simulink model "lab-6-simulink"  (R2018a)
settings: Solver=ode23t  StartTime=0.0  StopTime=10.0  RelTol=1e-3
values from neighbouring files (symbols this model uses):
  Kd = 0    [lab-6-q1.m]    (also in lab-6-q2.m; lab-6-q3.m = 10)
  Ki = 0    [lab-6-q1.m]    (also in lab-6-q2.m = 15; lab-6-q3.m = 5)
  Kp = 40    [lab-6-q1.m]    (also in lab-6-q2.m = 5; lab-6-q3.m = 5)
libraries: simulink x1
settings Model: Creator=katherto  LastModifiedBy=katherto

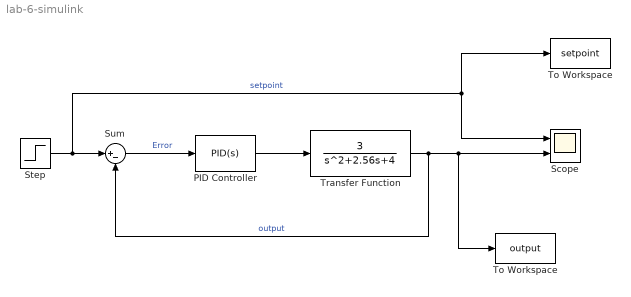
== system lab-6-simulink ==
  "PID Controller  " : simulink/Continuous/PID Controller  Controller=PID  TimeDomain=Continuous-time  SampleTime=-1  IntegratorMethod=Forward Euler  FilterMethod=Forward Euler  Form=Parallel  UseFilter=on  ControllerParametersSource=internal  P=Kp  I=Ki  D=Kd  N=100  InitialConditionSource=internal  InitialConditionForIntegrator=0  InitialConditionForFilter=0  ExternalReset=none  LimitOutput=off  UpperSaturationLimit=inf  LowerSaturationLimit=-inf  LinearizeAsGain=on  AntiWindupMode=none  Kb=1  TrackingMode=off  Kt=1  PParamMin=[]  PParamMax=[]  IParamMin=[]  IParamMax=[]  DParamMin=[]  DParamMax=[]  NParamMin=[]  NParamMax=[]  KbParamMin=[]  KbParamMax=[]  KtParamMin=[]  KtParamMax=[]  POutMin=[]  POutMax=[]  IOutMin=[]  IOutMax=[]  DOutMin=[]  DOutMax=[]  NOutMin=[]  NOutMax=[]  KbOutMin=[]  KbOutMax=[]  KtOutMin=[]  KtOutMax=[]  IntegratorOutMin=[]  IntegratorOutMax=[]  FilterOutMin=[]  FilterOutMax=[]  SumOutMin=[]  SumOutMax=[]  SumI1OutMin=[]  SumI1OutMax=[]  SumI2OutMin=[]  SumI2OutMax=[]  SumI3OutMin=[]  SumI3OutMax=[]  SumDOutMin=[]  SumDOutMax=[]  SaturationOutMin=[]  SaturationOutMax=[]  IntegratorContinuousStateAttributes=''  IntegratorStateMustResolveToSignalObject=off  IntegratorRTWStateStorageClass=Auto  FilterContinuousStateAttributes=''  FilterStateMustResolveToSignalObject=off  FilterRTWStateStorageClass=Auto  DifferentiatorICPrevScaledInput=0  DifferentiatorOutMin=[]  DifferentiatorOutMax=[]  FilterDiffOutCoefMin=[]  FilterDiffOutCoefMax=[]  SumDenOutMin=[]  SumDenOutMax=[]  SumNumOutMin=[]  SumNumOutMax=[]  ReciprocalOutMin=[]  ReciprocalOutMax=[]  DivideOutMin=[]  DivideOutMax=[]  TunerSelectOption=Transfer Function Based (PID Tuner App)
  "Scope  " : Scope  NumInputPorts=2
  "Step  " : Step  Time=0  After=5  SampleTime=0
  Sum : Sum  Inputs=|+-
  "To Workspace " : ToWorkspace  VariableName=output  SaveFormat=Timeseries  SampleTime=-1
  "To Workspace  " : ToWorkspace  VariableName=setpoint  SaveFormat=Timeseries  SampleTime=-1
  Transfer Function : TransferFcn  Numerator=[3]  Denominator=[1 2.56 4]
  wires:
  "Step  "/1 -> "To Workspace  "/1, "Scope  "/1, Sum/1  "setpoint"
  Sum/1 -> "PID Controller  "/1  "Error"
  "PID Controller  "/1 -> Transfer Function/1
  Transfer Function/1 -> Sum/2, "To Workspace "/1, "Scope  "/2  "output"
